simulink model "Signal_Demixer"  (R2022b)
settings: Solver=FixedStepAuto  StartTime=0.0  StopTime=10  FixedStep=1/Fs  RelTol=1e-3
values from neighbouring files (symbols this model uses):
  alpha_AC_d = alpha_AC    (= 1)    [basic.m]
  alpha_AD_d = alpha_AD    (= 1)    [basic.m]
  alpha_BC_d = alpha_BC    (= 1)    [basic.m]
  alpha_BD_d = alpha_BD    (= 1)    [basic.m]
  beta_AC_d = beta_AC + ceil(shift*2*(rand-.5))    [basic.m]
  beta_AD_d = beta_AD + ceil(shift*2*(rand-.5))    [basic.m]
  beta_BC_d = beta_BC + ceil(shift*2*(rand-.5))    [basic.m]
  beta_BD_d = beta_BD + ceil(shift*2*(rand-.5))    [basic.m]
settings Model: Creator=yash2  LastModifiedBy=yash2
settings DebuggingCC: UnconnectedInputMsg=warning  UnconnectedOutputMsg=warning  UnconnectedLineMsg=warning
settings ModelReferenceCC: EnableRefExpFcnMdlSchedulingChecks=on
settings RTWCC: DLArmComputeVersion=19.05

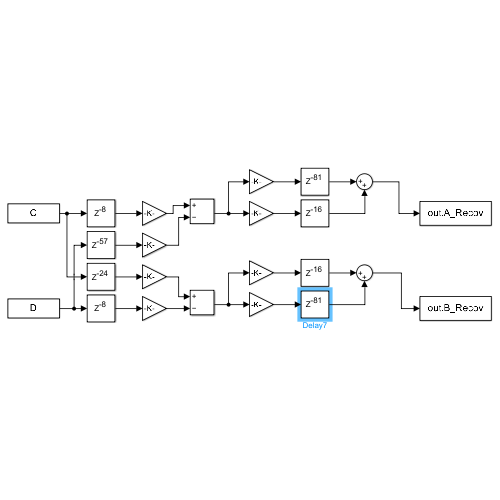
[thumbnail: Simulink's stored preview of the top-level diagram]
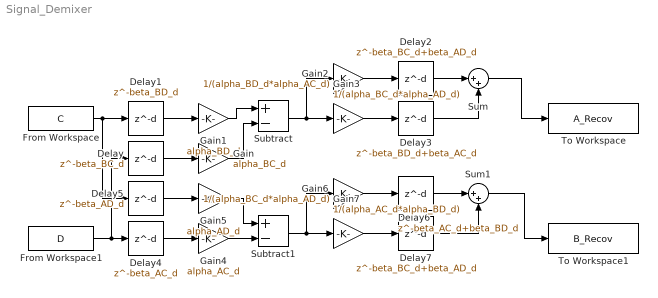
== system Signal_Demixer ==
  Delay : Delay  DelayLength=beta_BC_d  InitialCondition=0
  Delay1 : Delay  DelayLength=beta_BD_d  InitialCondition=0
  Delay2 : Delay  DelayLength=beta_BC_d+beta_AD_d  InitialCondition=0
  Delay3 : Delay  DelayLength=beta_BD_d+beta_AC_d  InitialCondition=0
  Delay4 : Delay  DelayLength=beta_AC_d  InitialCondition=0
  Delay5 : Delay  DelayLength=beta_AD_d  InitialCondition=0
  Delay6 : Delay  DelayLength=beta_AC_d+beta_BD_d  InitialCondition=0
  Delay7 : Delay  DelayLength=beta_BC_d+beta_AD_d  InitialCondition=0
  From Workspace : FromWorkspace  VariableName=C  OutputAfterFinalValue=Setting to zero
  From Workspace1 : FromWorkspace  VariableName=D  OutputAfterFinalValue=Setting to zero
  Gain : Gain  Gain=alpha_BC_d
  Gain1 : Gain  Gain=alpha_BD_d
  Gain2 : Gain  Gain=1/(alpha_BD_d*alpha_AC_d)
  Gain3 : Gain  Gain=1/(alpha_BC_d*alpha_AD_d)
  Gain4 : Gain  Gain=alpha_AC_d
  Gain5 : Gain  Gain=alpha_AD_d
  Gain6 : Gain  Gain=1/(alpha_BC_d*alpha_AD_d)
  Gain7 : Gain  Gain=1/(alpha_AC_d*alpha_BD_d)
  Subtract : Sum  Inputs=+-
  Subtract1 : Sum  Inputs=+-
  Sum : Sum  Inputs=|++
  Sum1 : Sum  Inputs=|++
  To Workspace : ToWorkspace  VariableName=A_Recov  SampleTime=-1
      settings: Save2DSignal=2-D array (concatenate along first dimension)
  To Workspace1 : ToWorkspace  VariableName=B_Recov  SampleTime=-1
      settings: Save2DSignal=2-D array (concatenate along first dimension)
  wires:
  Delay/1 -> Gain/1
  From Workspace1/1 -> Delay4/1, Delay/1
  Gain/1 -> Subtract/2
  From Workspace/1 -> Delay5/1, Delay1/1
  Delay1/1 -> Gain1/1
  Gain1/1 -> Subtract/1
  Sum/1 -> To Workspace/1
  Subtract/1 -> Gain3/1, Gain2/1
  Gain2/1 -> Delay2/1
  Delay2/1 -> Sum/1
  Delay3/1 -> Sum/2
  Gain3/1 -> Delay3/1
  Delay4/1 -> Gain4/1
  Gain4/1 -> Subtract1/2
  Delay5/1 -> Gain5/1
  Gain5/1 -> Subtract1/1
  Gain7/1 -> Delay7/1
  Sum1/1 -> To Workspace1/1
  Gain6/1 -> Delay6/1
  Delay7/1 -> Sum1/2
  Delay6/1 -> Sum1/1
  Subtract1/1 -> Gain7/1, Gain6/1
